simulink model "control_sorat_germ"  (Simulink 7.8)
settings: Solver=ode45  StartTime=0.0  StopTime=70  RelTol=1e-3
settings Model: Creator=nike  LastModifiedBy=nike

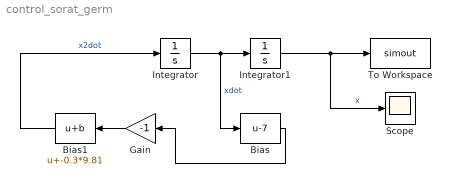
== system control_sorat_germ ==
  Bias : Bias  Bias=-7
  Bias1 : Bias  Bias=-0.3*9.81
  Gain : Gain  Gain=-1
  Integrator : Integrator  InitialCondition=70
  Integrator1 : Integrator
  Scope : Scope
  To Workspace : ToWorkspace  VariableName=simout  SampleTime=-1  SaveFormat=Structure
  wires:
  Integrator/1 -> Integrator1/1, Bias/1  "xdot"
  Integrator1/1 -> To Workspace/1, Scope/1  "x"
  Bias1/1 -> Integrator/1  "x2dot"
  Bias/1 -> Gain/1
  Gain/1 -> Bias1/1
